simulink model "State_Space_Simulation_LQI"  (R2019a)
settings: Solver=VariableStepAuto  StartTime=0.0  StopTime=10  RelTol=1e-3
values from neighbouring files (symbols this model uses):
  A = 1/5    (= 0.2)    [Pendulum_SS_Init.m]    (also in Pendulum_State_Space.m = [0, 1; -b, -a])
  b = 36.29    [Pendelum_TF2.mat]
  B = [0, c]'    [Pendulum_State_Space.m]
  c = 20.51    [Pendelum_TF2.mat]
  C = eye(2)    [Pendulum_State_Space.m]
  G = [1, 0]'    [Pendulum_State_Space.m]
  K = K_joint(1:2)    [Pendulum_State_Space.m]
  Ki = -K_joint(3)    [Pendulum_State_Space.m]
settings Model: Creator=QuarcUser  LastModifiedBy=QuarcUser

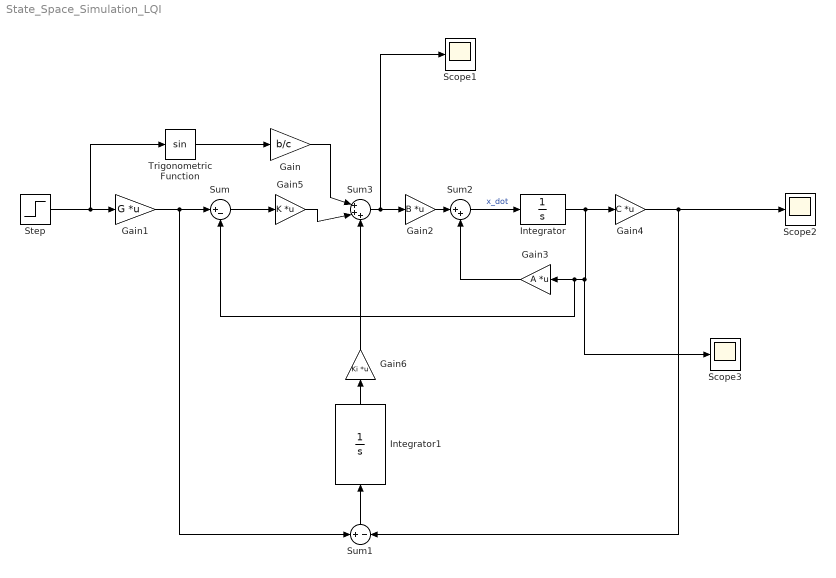
== system State_Space_Simulation_LQI ==
  Gain : Gain  Gain=b/c
  Gain1 : Gain  Gain=G  Multiplication=Matrix(K*u)
  Gain2 : Gain  Gain=B  Multiplication=Matrix(K*u)
  Gain3 : Gain  Gain=A  Multiplication=Matrix(K*u)
  Gain4 : Gain  Gain=C  Multiplication=Matrix(K*u)
  Gain5 : Gain  Gain=K  Multiplication=Matrix(K*u)
  Gain6 : Gain  Gain=Ki  Multiplication=Matrix(K*u)
  Integrator : Integrator  InitialCondition=[0;0]
  Integrator1 : Integrator  InitialCondition=[0;0]
  Scope1 : Scope
  Scope2 : Scope
  Scope3 : Scope
  Step : Step  SampleTime=.002
  Sum : Sum  Inputs=|+-
  Sum1 : Sum  Inputs=+-
  Sum2 : Sum  Inputs=|++
  Sum3 : Sum  Inputs=|+++
  Trigonometric Function : Trigonometry
  wires:
  Sum/1 -> Gain5/1
  Gain2/1 -> Sum2/1
  Sum2/1 -> Integrator/1  "x_dot"
  Gain3/1 -> Sum2/2
  Sum1/1 -> Integrator1/1
  Gain4/1 -> Sum1/2, Scope2/1
  Integrator1/1 -> Gain6/1
  Integrator/1 -> Scope3/1, Gain3/1, Sum/2, Gain4/1
  Gain1/1 -> Sum1/1, Sum/1
  Step/1 -> Trigonometric Function/1, Gain1/1
  Gain/1 -> Sum3/1
  Sum3/1 -> Scope1/1, Gain2/1
  Gain5/1 -> Sum3/2
  Gain6/1 -> Sum3/3
  Trigonometric Function/1 -> Gain/1
